simulink model "tutorial5"  (Simulink 2.20)
settings: Solver=ode5  StartTime=0.0  StopTime=tstop  FixedStep=tstep  MaxStep=tstep  RelTol=1e-3  AbsTol=1e-3
settings Model: SaveTime=off  SaveOutput=off  ConsistencyChecking=off  RTWPlaceOutputsASAP=off

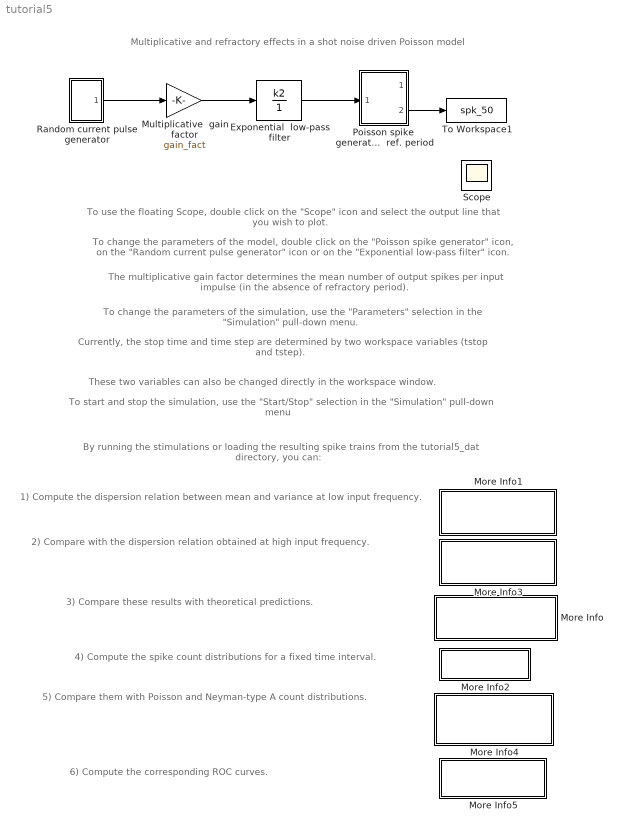
== system tutorial5 ==
  note: Multiplicative and refractory effects in a shot noise driven Poisson model
  note: To use the floating Scope, double click on the "Scope" icon and select the output line
      | that you wish to plot.
  note: To change the parameters of the model, double click on the  "Poisson spike generator" icon,
      |  on the "Random current pulse generator" icon or on the "Exponential low-pass filter" icon.
  note: The multiplicative gain factor determines the mean number of output spikes per input impulse
      | (in the absence of refractory period).
  note: To change the parameters of the simulation, use the "Parameters" selection in the
      | "Simulation" pull-down menu.
  note: Currently, the stop time and time step are determined by two workspace variables
      | (tstop and tstep).
  note: These two variables can also be changed directly in the workspace window.
  note: To start and stop the simulation, use the "Start/Stop" selection in the "Simulation"
      | pull-down menu
  note: By running the stimulations or loading the resulting spike trains from the tutorial5_dat
      | directory, you can:
  note: 1) Compute the dispersion relation between mean and variance
      | at low input frequency.
  note: 2) Compare with the dispersion relation obtained at high
      | input frequency.
  note: 3) Compare these results with theoretical predictions.
  note: 4) Compute the spike count distributions for a fixed time interval.
  note: 5) Compare them with Poisson and Neyman-type A count
      | distributions.
  note: 6) Compute the corresponding ROC curves.
  Exponential  low-pass filter : DiscreteFilter  Numerator=k2  Denominator=1  SampleTime=dt  mask(Exponential low-pass filter){@1=27, @2=1024, @3=tstep}
      mask prompts: @1 "Time constant [msec]"; @2 "Number of  points"; @3 "time step [msec]"
      mask help: Parameters
      mask init:
      | tau = @1; n = @2; dt = @3; t = [0:1:n-1]*dt; k2 = exp(-t/tau) ; k2 = k2/norm(k2);
      mask Display: plot(t,k2);
  More Info : Subsystem
      mask Display: disp('Theoretical mean to\n variance dispersion')
  More Info1 : Subsystem
      mask Display: disp('Dispersion relation\nat low input\nfrequencies')
  More Info2 : Subsystem
      mask Display: disp('Spike count\ndistributions')
  More Info3 : Subsystem
      mask Display: disp('Dispersion relation\nat high input\nfrequencies')
  More Info4 : Subsystem
      mask Display: disp('NTA and Poisson\nspike count\ndistributions')
  More Info5 : Subsystem
      mask Display: disp('ROC curves')
  Multiplicative  gain factor : Gain  Gain=gain_fact  mask(Multiplicative gain factor){@1=2, @2=27, @3=1024, @4=tstep, @5=10, @6=.5}
      mask prompts: @1 "Multiplication factor"; @2 "Filter time constant [msec]"; @3 "Number of points"; @4 "time step [msec]"; @5 "mean threshold [mV]"; @6 "Capacitance [nF]"
      mask help: Parameters
      mask init:
      | k2 = exp(-(0:@3-1)*@4/@2); k2 = k2/norm(k2); hbar = sum(k2);gain_fact = @5*@6*@1/(@4*hbar);
      mask Help: This block computes the multiplicative factor with which a shot noise  pulse should be multiplied to implement a given multiplicative gain for shot noise cascaded through an exponential filter and a Poisson pulse generator.
      mask Display: disp('alpha')
  Poisson spike  generator with  ref. period : Subsystem  mask(I&F p. thres., ref. per.){@1=tstep, @2=10, @3=.5, @4=2}
      mask prompts: @1 "time step [msec]"; @2 "mean threshold [mV]"; @3 "Capacitance [nF]"; @4 "refractory period [msec]"
      mask help: Parameters
      mask init:
      | dt = @1; thres = @2; C = @3; ref = @4;
      mask Help: For a detailled description of the model, please type 'help piandfr' in the main matlab window
      mask Display: disp('Vm \n\n spikes')
  Random current pulse generator : Subsystem  mask(Pulse generator){@1=tstep, @2=0, @3=50, @4=tstep, @5=1}
      mask prompts: @1 "time step [msec]"; @2 "start time [msec]"; @3 "period [msec]"; @4 "width [msec]"; @5 "pulse height [nA]"
      mask help: Parameters:
      mask init:
      | dt = @1; s = @2; p = @3; w = @4; h = @5;
      mask Help: Pulse generator, for a detailled description of the model, type 'help pulsegen' in the main matlab window
      mask Display: plot(0,0,100,100,[90,75,75,60,60,35,35,20,20,10],[20,20,80,80,20,20,80,80,20,20])
  Scope : Scope
      settings: TickLabels=on  TimeRange=500.000000  YMin=-2.000000  YMax=2.000000  SaveToWorkspace=off  SaveName=ScopeData
  To Workspace1 : ToWorkspace  VariableName=spk_50  SampleTime=0
      settings: Buffer=ceil(tstop/tstep)
  wires:
  Random current pulse generator/1(out_1) -> Multiplicative  gain factor/1
  Multiplicative  gain factor/1 -> Exponential  low-pass filter/1
  Exponential  low-pass filter/1 -> Poisson spike  generator with  ref. period/1(in_1)
  Poisson spike  generator with  ref. period/2(out_1) -> To Workspace1/1

== system tutorial5/More Info ==
  note: sndpdisp(50,2,27,2,10,500,10)
  note: in the workspace window.
  note: The parameters are:
  note: 50 = rate of the input pulses (in Hz).
  note: 2 = multiplication parameter.
  note: 27 = low-pass filter time constant (msec).
  note: 2 = refractory period (msec).
  note: 10 = smallest interval on which the mean and
      |       variance should be computed (in msec).
  note: 500 = largest interval (in msec)
  note: 10 = interval increment (in msec).
  note: To compute the theoretical mean to
      | variance dispersions, enter:
  note: Similarly, enter:
  note: sndpdisp(20,2,27,2,20,1000,20)

== system tutorial5/More Info1 ==
  note: To compute the mean to variance dispersion at
      | low stimulus frequencies, run the simulation or load
      | the resulting output spike train by entering:
  note: load tutorial5_dat/spk_50
  note: in the workspace window. Then enter:
  note: dispersion(spk_50,tstep,20,1000,20)
  note: tstep = time step for the simulation
  note: The parameters are:
  note: spk_50 = output spike train
  note: 20 = smallest interval on which the mean and
      |       variance should be computed (in msec).
  note: 1000 = largest interval (in msec)
  note: 20 = interval increment (in msec).

== system tutorial5/More Info2 ==
  note: To plot the spike count distributions, enter
  note: countprob(spk_20,250,40,tstep)
  note: in the workspace window. The parameters are:
  note: spk_20 = spike train:
  note: 250 = time interval (msec)
  note: 40 = maximal spike count
  note: tstep = time step for the simulation (in msec).
  note: Similarly, enter:
  note: countprob(spk_50,250,40,tstep)1
  note: hold on

== system tutorial5/More Info3 ==
  note: To compute the mean to variance dispersion at
      | high stimulus frequencies, proceed as follows:
  note: 1) Double click on the "Random current pulse generator"
      | icon and modify the mean period between pulses to 20
      | msec. Similarly, change the name of the output variable
      | to spk_20 and then run the simulation.
  note: Alternatively, load the result of the simulation by typing:
  note: in the workspace window. Then enter:
  note: load tutorial5_dat/spk_20
  note: 10 = interval increment (in msec).
  note: 500 = largest interval (in msec)
  note: 10 = smallest interval on which the mean and
      |       variance should be computed (in msec).
  note: tstep = time step for the simulation
  note: spk_20 = output spike train
  note: The parameters are:
  note: dispersion(spk_20,tstep,10,500,10)
  note: hold on

== system tutorial5/More Info4 ==
  note: in the workspace window. The parameters are:
  note: 8.35 = mean spike count.
  note: To plot the corresponding NTA spike count
      | distributions, enter
  note: neymtacnt(8.35,2.45-1,40)
  note: 40 = maximal spike count.
  note: Similarly, enter:
  note: neymtacnt(19.7,1.78-1,40)
  note: To plot the corresponding Poisson spike count
      | distributions, enter:
  note: in the workspace window. The parameters are:
  note: 2.45-1 = effective multiplication parameter (given by
      | the dispersion minus 1).
  note: poisscnt(8.35/250e-3,250,40)
  note: 250 = time interval (in msec).
  note: 8.35/250e-3 = mean rate of the Poisson process (in Hz).
  note: 40 = maximal spike count.
  note: Similarly, enter:
  note: poisscnt(19.7/250e-3,250,40)

== system tutorial5/More Info5 ==
  note: To plot the corresponding ROC curves, enter
  note: [cnt,prb1] = countprob(spk_50,250,40,tstep);
  note: [cnt,prb2] = countprob(spk_20,250,40,tstep);
  note: roc(cnt,prb1,prb2)
  note: [cnt, nta1] = neymtacnt(8.35,2.45-1,40);
  note: [cnt, nta2] = neymtacnt(19.7,1.78-1,40);
  note: hold on; subplot(2,1,1); hold on;
  note: roc(cnt,nta1,nta2)
  note: [cnt, poi1] = poisscnt(8.35/250e-3,250,40);
  note: [cnt, poi2] = poisscnt(19.7/250e-3,250,40);
  note: roc(cnt,poi1,poi2)
  note: in the workspace window.
  note: To compare the experimental roc curve with the
      | corresponding gaussian roc curve enter:
  note: [pds, pfs] = roc(cnt,prb1,prb2);
  note: [pdg, pfg] = roc(8.35,4.52,19.7,5.93)
  note: figure(5); plot(pfs,pds,pfg,pdg,'g');
  note: in the workspace window.

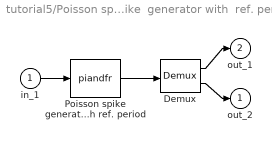
== system tutorial5/Poisson spike  generator with  ref. period ==
  in_1 : Inport  Port=1  PortWidth=-1  SampleTime=-1
  Demux : Demux  Outputs=2
  Poisson spike generator with ref. period : S-Function  FunctionName=piandfr  Parameters=dt,thres,C, ref  PortCounts=[]  SFunctionModules=''
  out_2 : Outport  Port=1  InitialOutput=0
  out_1 : Outport  Port=2  InitialOutput=0
  wires:
  in_1/1 -> Poisson spike generator with ref. period/1
  Demux/2 -> out_2/1
  Demux/1 -> out_1/1
  Poisson spike generator with ref. period/1 -> Demux/1

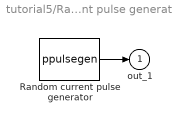
== system tutorial5/Random current pulse generator ==
  Random current pulse generator : S-Function  FunctionName=ppulsegen  Parameters=dt,s,p,w,h  PortCounts=[]  SFunctionModules=''
  out_1 : Outport  Port=1  InitialOutput=0
  wires:
  Random current pulse generator/1 -> out_1/1
